simulink subsystem "PD_roll"  (R2021a)
settings: Solver=VariableStepAuto  StartTime=0.0  StopTime=10.0  RelTol=1e-3
undefined symbols (not defined in the file): Tmax
libraries: simulink x1, vrlib x1
settings Model: Creator=Laura  LastModifiedBy=Laura

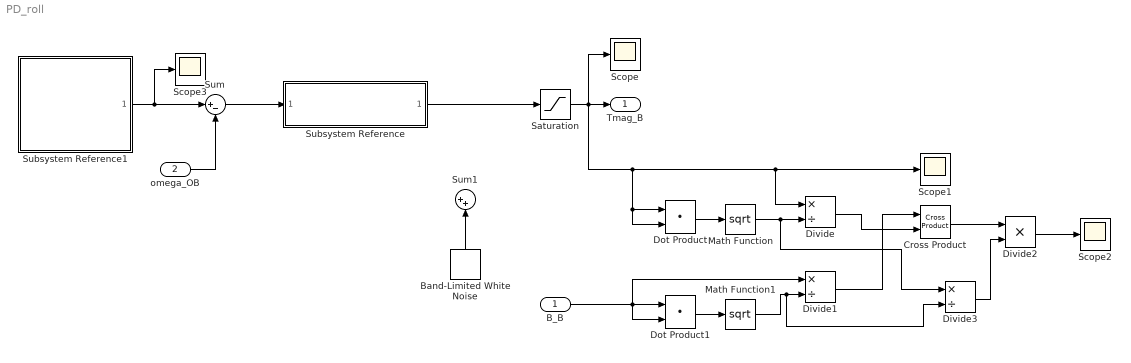
== system PD_roll ==
  B_B : Inport
  "omega_OB " : Inport  Port=2
  Band-Limited White Noise : simulink/Sources/Band-Limited White Noise  Cov=[0.000000005*Tmax]  Ts=0.1  seed=[23341]
  Cross Product : vrlib/Utilities/Cross Product
  Divide : Product  Inputs=*/
  Divide1 : Product  Inputs=*/
  Divide2 : Product  Inputs=**
  Divide3 : Product  Inputs=*/
  Dot Product : DotProduct  InputSameDT=on  OutDataTypeStr=Inherit: Inherit via internal rule
  Dot Product1 : DotProduct  InputSameDT=on  OutDataTypeStr=Inherit: Inherit via internal rule
  Math Function : Math  Operator=sqrt  SignedPower=on  SaturateOnIntegerOverflow=on
  Math Function1 : Math  Operator=sqrt  SignedPower=on  SaturateOnIntegerOverflow=on
  Saturation : Saturate  UpperLimit=Tmax  LowerLimit=-Tmax
  Scope{,1..3} (4 alike) : Scope
  Subsystem Reference : Subsystem  ReferencedSubsystem=PID
  Subsystem Reference1 : Subsystem  ReferencedSubsystem=Maneuver
  Sum : Sum  Inputs=|+-
  Sum1 : Sum  Inputs=|++
  Tmag_B : Outport
  wires:
  Subsystem Reference1/1 -> Sum/1, Scope3/1
  "omega_OB "/1 -> Sum/2
  Sum/1 -> Subsystem Reference/1
  Saturation/1 -> Scope1/1, Divide/1, Dot Product/1, Dot Product/2, Tmag_B/1, Scope/1
  Dot Product/1 -> Math Function/1
  Dot Product1/1 -> Math Function1/1
  B_B/1 -> Dot Product1/1, Dot Product1/2, Divide1/1
  Math Function/1 -> Divide/2, Divide3/1
  Math Function1/1 -> Divide1/2, Divide3/2
  Divide/1 -> Cross Product/2
  Divide1/1 -> Cross Product/1
  Cross Product/1 -> Divide2/1
  Divide3/1 -> Divide2/2
  Divide2/1 -> Scope2/1
  Subsystem Reference/1 -> Saturation/1
  ? -> Sum1/1
  Band-Limited White Noise/1 -> Sum1/2
